simulink model "Exercise4"  (Simulink 6.1)
settings: Solver=ode45  StartTime=0.0  StopTime=10.0  RelTol=1e-3
libraries: simulink x1
settings Model: LastModifiedBy=Inderjot
settings DebuggingCC: SolverPrmCheckMsg=warning

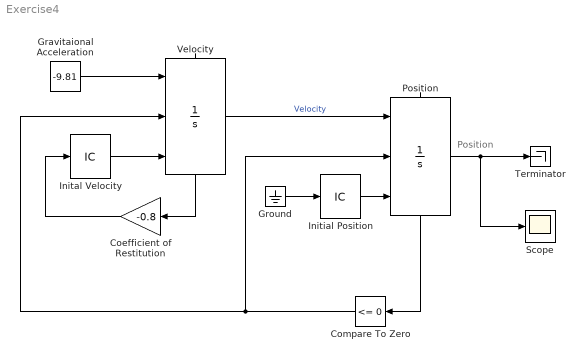
== system Exercise4 ==
  note: Position
  Coefficient of Restitution : Gain  Orientation=left  Gain=-0.8
  Compare To Zero : simulink/Logic and Bit Operations/Compare To Zero  Orientation=left  relop=<=  LogicOutDataTypeMode=boolean  ZeroCross=off
  Gravitaional Acceleration : Constant  Value=-9.81
  Ground : Ground
  Inital Velocity : InitialCondition  Value=15
  Initial Position : InitialCondition  Value=10
  Position : Integrator  ExternalReset=rising  InitialConditionSource=external  LimitOutput=on  ShowStatePort=on
  Scope : Scope
  Terminator : Terminator
  Velocity : Integrator  ExternalReset=rising  InitialConditionSource=external  ShowStatePort=on
  wires:
  Gravitaional Acceleration/1 -> Velocity/1
  Velocity/1 -> Position/1  "Velocity"
  Velocity/State -> Coefficient of Restitution/1
  Inital Velocity/1 -> Velocity/3
  Coefficient of Restitution/1 -> Inital Velocity/1
  Position/State -> Compare To Zero/1
  Compare To Zero/1 -> Velocity/2, Position/2
  Initial Position/1 -> Position/3
  Ground/1 -> Initial Position/1
  Position/1 -> Terminator/1, Scope/1
